simulink model "full_Model"  (R2023b)
settings: Solver=ode15s  StartTime=0.0  StopTime=200  RelTol=1e-3
InitFcn:
  | clear all
  | clc
  | 
  | load('EnvironmentData.mat')
  | load('userMap.mat')
  | 
  | starty = 1;
  | startx = 1;
  | endy = 20;
  | endx = 20;
  | objy = [];
  | objx = [];
  | bally = 11;
  | ballx = 11;
  | 
  | objPos=[objx,objy];
  | ballPos=[11,11,0.54];
  | boxPos=[];
  | 
  | ManipulatorSetup
  | init_quad_new_leg_raibert_strategy_v2
  | transitionMode = [-1];
values from neighbouring files (symbols this model uses):
  body = rigidBody('tool')    [InverseKinematicsV2.m]
  tar1Len = 9    [EnvironmentData.mat]
  target = [1 2.44274045536 4.0666557818 4.62742644863 6.44502800895 8.36141317519 9.41392894318 10.3865588461 10.4 10.4 11.7644392896 13.2870590067 ... (34 elements, 17x2)]    [EnvironmentData.mat]
  tarLen = 17    [EnvironmentData.mat]
undefined symbols (not defined in the file or in its folder): planner
libraries: sim3dlib x33, sharedtransform x2, visionsinks x1, visionanalysis x1, visiongeotforms x1, sim3dcameralib x1
(part 3 of 7)

== stateflow chart full_Model/Controller/High Level Mode Stateflow ==
  state ResetPos
    mode=0;
    ManipTask=1;
  state Stationary
    mode=0;
    ManipTask=0;
  state Turning_Right
    mode=2;
  state Walking
    mode=1;
  state Turning_Left
    mode=3;
  Turning_Right -> ResetPos [order 2] : [resetPos==1]{pos_index=pos_index+2}
  Stationary -> ResetPos [order 2] : [resetPos==1]{pos_index=pos_index+2}
  ResetPos -> Stationary : [manipState==5]
  Walking -> ResetPos [order 4] : [resetPos==1]{pos_index=pos_index+2}
  Turning_Left -> ResetPos [order 2] : [resetPos==1]{pos_index=pos_index+2}
  (default) -> Stationary : {pos_index =2 }
  Turning_Left -> Stationary [order 1] : [delta_theta < ang_threshold]
  Turning_Right -> Stationary [order 1] : [delta_theta > -ang_threshold]
  Stationary -> Walking [order 1] : [~target_reached]
  Walking -> Stationary [order 3] : [target_reached]
      | {pos_index = pos_index + 1}
  Walking -> Turning_Right [order 2] : [delta_theta < -ang_threshold]
  Walking -> Turning_Left [order 1] : [delta_theta > ang_threshold]
  data: pos_index output =0; mode output =0; target_reached input; delta_theta input; ang_threshold local =0.2; resetPos input; ManipTask output; manipState input

== stateflow chart full_Model/Controller/Chart ==
  state PathFollowing
    resetPos=0;
  state ManipulatorTask
    resetPos=1;
  (default) -> PathFollowing
  PathFollowing -> ManipulatorTask : [pos_index==tar1Len]
  ManipulatorTask -> PathFollowing : [manipState==5]
  data: pos_index input; tar1Len input; resetPos output; manipState input

== matlab function full_Model/TNR Annotation ==
  data: Area input; bboxes input size=[20 4]; scores input size=[20  1]; In input; In output
function In = TNRAnnotation(Area, bboxes, scores, In)

if ~isempty(bboxes)
    In = insertObjectAnnotation(In, 'rectangle',bboxes,scores);
    
end
In = insertObjectAnnotation(In, 'rectangle',Area,'.');
end

== matlab function full_Model/TNR Annotation1 ==
  data: bboxes input size=[20 4]; Output output; Area input
function Output = VisionOutput(bboxes, Area)
bbheight = height(bboxes);
xmin = Area(1);
xmax = Area(1) + Area(3);
ymin = Area(2);




%% first if statement decides whether we need to turn on not 
if bbheight == 1 
    if ((bboxes(1,1) + (bboxes(1,3)/2))  > xmin && (bboxes(1,1) + (bboxes(1,3)/2)) < xmax  && (bboxes(1,2) + bboxes(1,4)) > ymin)
        Turn = 1;
    else
        Turn = 0;
    end
elseif bbheight == 2
     if ((bboxes(1,1) + (bboxes(1,3)/2))  > xmin && (bboxes(1,1) + (bboxes(1,3)/2)) < xmax  && (bboxes(1,2) + bboxes(1,4)) > ymin ) || ...
        ((bboxes(2,1) + (bboxes(2,3)/2))  > xmin && (bboxes(2,1) + (bboxes(2,3)/2)) < xmax  && (bboxes(2,2) + bboxes(2,4)) > ymin )
        Turn = 1;
     else
        Turn = 0;
     end
elseif bbheight == 3
    if ((bboxes(1,1) + (bboxes(1,3)/2))  > xmin && (bboxes(1,1) + (bboxes(1,3)/2)) < xmax  && (bboxes(1,2) + bboxes(1,4)) > ymin ) || ...
       ((bboxes(2,1) + (bboxes(2,3)/2))  > xmin && (bboxes(2,1) + (bboxes(2,3)/2)) < xmax  && (bboxes(2,2) + bboxes(2,4)) > ymin ) || ...
       ((bboxes(3,1) + (bboxes(3,3)/2))  > xmin && (bboxes(3,1) + (bboxes(3,3)/2)) < xmax  && (bboxes(3,2) + bboxes(3,4)) > ymin )
        Turn = 1;
    else
        Turn = 0;
    end
elseif bbheight == 4
    if ((bboxes(1,1) + (bboxes(1,3)/2))  > xmin && (bboxes(1,1) + (bboxes(1,3)/2)) < xmax  && (bboxes(1,2) + bboxes(1,4)) > ymin ) || ...
       ((bboxes(2,1) + (bboxes(2,3)/2))  > xmin && (bboxes(2,1) + (bboxes(2,3)/2)) < xmax  && (bboxes(2,2) + bboxes(2,4)) > ymin ) || ...
       ((bboxes(3,1) + (bboxes(3,3)/2))  > xmin && (bboxes(3,1) + (bboxes(3,3)/2)) < xmax  && (bboxes(3,2) + bboxes(3,4)) > ymin ) || ...
       ((bboxes(4,1) + (bboxes(4,3)/2))  > xmin && (bboxes(4,1) + (bboxes(4,3)/2)) < xmax  && (bboxes(4,2) + bboxes(4,4)) > ymin )
        Turn = 1;
    else
        Turn = 0;
    end
elseif bbheight == 5    
    if ((bboxes(1,1) + (bboxes(1,3)/2))  > xmin && (bboxes(1,1) + (bboxes(1,3)/2)) < xmax  && (bboxes(1,2) + bboxes(1,4)) > ymin ) || ...
       ((bboxes(2,1) + (bboxes(2,3)/2))  > xmin && (bboxes(2,1) + (bboxes(2,3)/2)) < xmax  && (bboxes(2,2) + bboxes(2,4)) > ymin ) || ...
       ((bboxes(3,1) + (bboxes(3,3)/2))  > xmin && (bboxes(3,1) + (bboxes(3,3)/2)) < xmax  && (bboxes(3,2) + bboxes(3,4)) > ymin ) || ...
       ((bboxes(4,1) + (bboxes(4,3)/2))  > xmin && (bboxes(4,1) + (bboxes(4,3)/2)) < xmax  && (bboxes(4,2) + bboxes(4,4)) > ymin ) || ...
       ((bboxes(5,1) + (bboxes(5,3)/2))  > xmin && (bboxes(5,1) + (bboxes(5,3)/2)) < xmax  && (bboxes(5,2) + bboxes(5,4)) > ymin )
        Turn = 1 ;
    else
        Turn = 0 ;
    end
else
    Turn = 0;
end
%% next statement decideshow many objects are to the left and right of the viewpoint
left = 0;
right = 0;

if Turn == 0
    Output = 1;
elseif Turn == 1
    for i = 1:1:bbheight
        if (bboxes(i,1) + (bboxes(i,3)/2)) < 112
            left = left + 1;
        elseif (bboxes(i,1) + (bboxes(i,3)/2)) >= 112
            right = right + 1;
        else
            Output = 1;
        end

    end
else
    Output = 0;
end
%% final statemnet suggests which way to turn
if Turn == 1 && left >= right
    Output = 3;
elseif Turn == 1 && left < right
    Output = 2;
else
    Output = 1;
end

== matlab function full_Model/Balancing ==
  data: FLpos input; y output; FRpos input; RLpos input; RRpos input; FLang input; FRang input; RLang input; RRang input; linkLen input; linkWeight input; footStates input
function y = balancing(FLpos, FRpos, RLpos, RRpos, FLang, FRang, RLang, RRang, linkLen, linkWeight, footStates)

inputMatrix = [ % Input Parameters
    5, 3, 2, 78, 35, -4;   
    5, 9, 2, 85, 53, 1;   
    22, 3, 4, 78, 35, -4; 
    22, 9, 4, 85, 53, 1;  
    5, 5, 0, 0, 0, 4; ];

baseWeight = 10;
link_weight_per_length = 0.5;

combinedPositions = calculateAdjustedEndpoints(inputMatrix); % Calling Function
result = calculateMidpoints(combinedPositions, link_weight_per_length, baseWeight);
centerOfMass = calculateCenterOfMass(result);

intersect = checkPlaneIntersection(combinedPositions, inputMatrix, centerOfMass);
visualizePlaneAndLine(combinedPositions, inputMatrix, centerOfMass);

figure; hold on; colors = ['r', 'g', 'b', 'k'];


for i = 1:4 % Plotting individual positions
    positions = combinedPositions((i-1)*3+1:i*3, :);
    scatter3(positions(:, 1), positions(:, 2), positions(:, 3), 36, colors(i), 'filled');
    plot3(positions(:, 1), positions(:, 2), positions(:, 3), colors(i));
end

scatter3(centerOfMass(1),centerOfMass(2),centerOfMass(3));

% Plotting connecting lines using combinedPositions
plot3([combinedPositions(3, 1), combinedPositions(6, 1)], [combinedPositions(3, 2), combinedPositions(6, 2)], [combinedPositions(3, 3), combinedPositions(6, 3)], 'm--', 'LineWidth', 2);
plot3([combinedPositions(3, 1), combinedPositions(9, 1)], [combinedPositions(3, 2), combinedPositions(9, 2)], [combinedPositions(3, 3), combinedPositions(9, 3)], 'm--', 'LineWidth', 2);
plot3([combinedPositions(12, 1), combinedPositions(6, 1)], [combinedPositions(12, 2), combinedPositions(6, 2)], [combinedPositions(12, 3), combinedPositions(6, 3)], 'c--', 'LineWidth', 2);
plot3([combinedPositions(12, 1), combinedPositions(9, 1)], [combinedPositions(12, 2), combinedPositions(9, 2)], [combinedPositions(12, 3), combinedPositions(9, 3)], 'c--', 'LineWidth', 2);

xlabel('X'); ylabel('Y'); zlabel('Z'); 
title('3D Plot of Combined Positions'); 
axis equal; grid on; view(3); hold off;

end


%% Functions

function combinedPositions = calculateAdjustedEndpoints(inputMatrix)
    combinedPositions = zeros(12, 3); % Initialize the output matrix
    for i = 1:4
        % Extract input parameters
        Foot = inputMatrix(i, 1:3);
        Ankle_Angle = inputMatrix(i, 4);
        Knee_Angle = inputMatrix(i, 5);
        Shoulder_angle = inputMatrix(i, 6);
        Link1_Length = inputMatrix(5, 1);
        Link2_Length = inputMatrix(5, 2);
        % Calculate the endpoints
        Link1_endpoint = zeros(1, 3);
        Link2_endpoint = zeros(1, 3);
        Link1_endpoint(1) = Foot(1) + Link1_Length * cos(deg2rad(Ankle_Angle));
        Link1_endpoint(2) = Foot(2);
        Link1_endpoint(3) = Foot(3) + Link1_Length * sin(deg2rad(Ankle_Angle));
        Link2_endpoint(1) = Link1_endpoint(1) + Link2_Length * cos(deg2rad(Knee_Angle));
        Link2_endpoint(2) = Link1_endpoint(2);
        Link2_endpoint(3) = Link1_endpoint(3) + Link2_Length * sin(deg2rad(Knee_Angle));
        % Adjust the endpoints based on the shoulder angle
        theta = deg2rad(Shoulder_angle);
        R = [1 0 0; 0 cos(theta) -sin(theta); 0 sin(theta) cos(theta)];
        Link1_endpoint_adjusted = R * (Link1_endpoint - Foot).' + Foot.';
        Link2_endpoint_adjusted = R * (Link2_endpoint - Foot).' + Foot.';
        % Assign the calculated positions to the output matrix
        startPos = (i-1)*3 + 1;
        combinedPositions(startPos:startPos+2, :) = [Foot; Link1_endpoint_adjusted.'; Link2_endpoint_adjusted.'];
    end
end

function outputMatrix = calculateMidpoints(inputMatrix, link_weight_per_length, baseWeight)
    outputMatrix = zeros(9, 4);     % Initialize the output matrix
    pointPairs = [1, 2; 2, 3; 4, 5; 5, 6; 7, 8; 8, 9; 10, 11; 11, 12]; % Define the pair
    for i = 1:size(pointPairs, 1)   % Calculate midpoint pos and link weight for each pair
        point1 = inputMatrix(pointPairs(i, 1), :);
        point2 = inputMatrix(pointPairs(i, 2), :);
        midpoint = (point1 + point2) / 2;
        distance = sqrt(sum((point1 - point2) .^ 2));
        weight = distance * link_weight_per_length;
        outputMatrix(i, 1:3) = midpoint;
        outputMatrix(i, 4) = weight;
    end
    centerPoints = mean(inputMatrix([3, 6, 9, 12], :), 1);  % Calculate base center
    outputMatrix(9, :) = [centerPoints, baseWeight];        % Add the baseWeight as its mass
end

function centerOfMass = calculateCenterOfMass(inputMatrix)
    % Initialize the variables for the sum of weighted coordinates and total mass
    weightedSum = [0, 0, 0];
    totalMass = 0;
    % Loop through each point
    for i = 1:size(inputMatrix, 1)
        % Extract the current point's coordinates and mass
        x = inputMatrix(i, 1);
        y = inputMatrix(i, 2);
        z = inputMatrix(i, 3);
        mass = inputMatrix(i, 4);
        % Update the weighted sum and total mass
        weightedSum = weightedSum + [x, y, z] * mass;
        totalMass = totalMass + mass;
    end
    % Calculate the center of mass coordinates
    centerOfMassCoordinates = weightedSum / totalMass;
    % Combine the center of mass coordinates with the total mass
    centerOfMass = [centerOfMassCoordinates, totalMass];
end

function intersect = checkPlaneIntersection(combinedPositions, inputMatrix, centerOfMass)
    % Determine which points to use from the combinedPositions matrix
    switch inputMatrix(5,6)
        case 1
            points = combinedPositions([6, 9, 12], :);
        case 2
            points = combinedPositions([3, 9, 12], :);
        case 3
            points = combinedPositions([3, 6, 12], :);
        case 4
            points = combinedPositions([3, 6, 9], :);
        otherwise
            error('Invalid input in inputMatrix(5,6)');
    end

    % Calculate the plane equation coefficients
    p1 = points(1, :);
    p2 = points(2, :);
    p3 = points(3, :);
    normal = cross(p2 - p1, p3 - p1);
    A = normal(1);
    B = normal(2);
    C = normal(3);
    D = -dot(normal, p1);

    % Check if the line from centerOfMass intersects the plane
    x0 = centerOfMass(1);
    y0 = centerOfMass(2);

    % If C is zero, the plane is parallel to the z-axis and can't intersect
    if C == 0
        intersect = 'NO';
        return;
    end

    % Find intersection point on the plane
    t = -(A * x0 + B * y0 + D) / C;
    intersectionPoint = [x0, y0, t];

    % Check if the intersection point is inside the triangle
    if isPointInTriangle(intersectionPoint, p1, p2, p3)
        intersect = 'YES';
    else
        intersect = 'NO';
    end
end

function inside = isPointInTriangle(pt, v1, v2, v3)
    % Barycentric coordinate system
    dX = pt(1) - v3(1);
    dY = pt(2) - v3(2);
    dX21 = v2(1) - v1(1);
    dY12 = v1(2) - v2(2);
    D = dY12 * (v3(1) - v1(1)) + dX21 * (v3(2) - v1(2));
    s = dY12 * dX + dX21 * dY;
    t = (v3(2) - v1(2)) * dX + (v1(1) - v3(1)) * dY;
    
    if D < 0
        inside = s <= 0 && t <= 0 && s + t >= D;
    else
        inside = s >= 0 && t >= 0 && s + t <= D;
    end
end


function visualizePlaneAndLine(combinedPositions, inputMatrix, centerOfMass)
    % Select points based on inputMatrix value
    switch inputMatrix(5,6)
        case 1
            points = combinedPositions([6, 9, 12], :);
        case 2
            points = combinedPositions([3, 9, 12], :);
        case 3
            points = combinedPositions([3, 6, 12], :);
        case 4
            points = combinedPositions([3, 6, 9], :);
        otherwise
            error('Invalid input in inputMatrix(5,6)');
    end

    % Plane calculation
    normal = cross(points(2,:) - points(1,:), points(3,:) - points(1,:));
    point = points(1,:);
    [xGrid, yGrid] = meshgrid(linspace(min(combinedPositions(:,1)), max(combinedPositions(:,1)), 10), ...
                             linspace(min(combinedPositions(:,2)), max(combinedPositions(:,2)), 10));
    zGrid = (-normal(1) * (xGrid - point(1)) - normal(2) * (yGrid - point(2)))/normal(3) + point(3);

    % Line calculation
    lineZ = linspace(min(zGrid(:)), max(zGrid(:)), 100);
    lineX = centerOfMass(1) * ones(size(lineZ));
    lineY = centerOfMass(2) * ones(size(lineZ));

    % Plotting
    figure;
    hold on;
    surf(xGrid, yGrid, zGrid, 'FaceAlpha', 0.5); % Draw plane
    plot3(lineX, lineY, lineZ, 'r', 'LineWidth', 2); % Draw line
    plot3(points(:,1), points(:,2), points(:,3), 'ko', 'MarkerSize', 10, 'MarkerFaceColor', 'k'); % Draw points
    xlabel('X');
    ylabel('Y');
    zlabel('Z');
    title('Visualization of Plane and Line');
    grid on;
    view(3);

    y = 0;
end

== matlab function full_Model/Controller/MATLAB Function1 ==
  settings: updateMethod=DISCRETE
  data: go input; mode output; targets input; tar1Len input; tarLen input; x input; y input; angle input; done output
function [mode,done] = broadside(go,targets,tar1Len,tarLen,x,y,angle)

persistent targetAssigned
if isempty(targetAssigned)
    targetAssigned=0;
end

persistent broadTarget
if isempty(broadTarget)
    broadTarget=[0,0];
end

persistent points
if isempty(points)
    points=0;
end

persistent point1
if isempty(point1)
    point1=[0,0];
end

persistent point2
if isempty(point2)
    point2=[0,0];
end

persistent currentTarget
if isempty(currentTarget)
    currentTarget=[0,0];
end


if go==1||go==2
    if targetAssigned==0
        if go==1
            broadTarget=targets(tar1Len,:);
        elseif go==2
            broadTarget=targets(tarLen,:);
        end
        if y>broadTarget(2)
            spacing=1;
        else
            spacing=-1;
        end
        if x>broadTarget(1)
            points=2;
            point1=[x,broadTarget(2)+spacing];
            point2=[broadTarget(1),broadTarget(2)+spacing];
        else
            points=1;
            point1=[broadTarget(1),broadTarget(2)+spacing];
        end
        currentTarget=point1;
        targetAssigned=1;
    end
    delta=currentTarget-[x,y];
    deltaDist=sqrt(delta(1).^2+delta(2).^2);
    targetAngle=atan2(delta(2),delta(1));
    deltaAngle=targetAngle-angle;
    if abs(deltaDist)>=0.2
        if deltaAngle<-0.1
            %disp('im left')
            %turn right
            mode=2;

        elseif deltaAngle>0.1
            %disp('im right')
            %turn left
            mode=3;
        else
            %disp('im forward')
            mode=1;
        end
        done=0;
    else
        if (currentTarget-point1)*[1;1]==0&&points==1
            currentTarget=[broadTarget(1),broadTarget(2)];
            done=0;
        elseif (currentTarget-point1)*[1;1]==0&&points==2
            currentTarget=point2;
            done=0;
        elseif (currentTarget-point2)*[1;1]==0
            currentTarget=[broadTarget(1),broadTarget(2)];
            done=0;
        else
            done=1;
        end
        mode=0;
    end
else
    targetAssigned=0;
    done=0;
    mode=0;
end

== stateflow chart full_Model/Controller/Task Controller/Task Controller Stateflow ==
  state PathFollowing
    endSim=false;
    resetPos=0;
    sqrt((target(tar1Len,1)-x).^2+ (target(tar1Len,2)-y).^2);
  state ManipulatorTask1
    resetPos=1;
  state PathFollowing2
    resetPos=0;
    sqrt((target(tar1Len,1)-x).^2+ (target(tar1Len,2)-y).^2);
  state ManipulatorTask2
    resetPos=2;
  state EndSim
    resetPos=0;
    endSim=true;
  PathFollowing -> ManipulatorTask1 : [sqrt((target(tar1Len,1)-x).^2+(target(tar1Len,2)-y).^2)<=1.5]{posToSkip=tar1Len-pos_index}
  (default) -> PathFollowing
  ManipulatorTask1 -> PathFollowing2 : [manipState>=5]
  PathFollowing2 -> ManipulatorTask2 : [sqrt((target(tarLen,1)-x).^2+ (target(tarLen,2)-y).^2)<=1.5]
  ManipulatorTask2 -> EndSim : [manipState>=11]
  data: tar1Len input; resetPos output; manipState input; tarLen input; endSim output; target input; y input; posToSkip output; x input; pos_index input

== stateflow chart full_Model/Controller/Path follower stateflow ==
  state Stationary1
    mode=0;
  state Walking1
    mode=1;
  state Turning_Left1
    mode=1;
  note: 0.35
  note: 1
  state ManipTask1
    ManipTask=1;
  state Broadside
    broadside=1;
  state Stationary
    mode=0;
  state ResetPos1
    mode=0;
  state Turning_Right
    mode=2;
  state Turning_Left
    mode=3;
  state Walking
    mode=1;
  state ManipTask2
    ManipTask=2;
  state ResetPos2
    mode=0;
  state Broadside1
    broadside=2;
  Walking1 -> Turning_Left1 : [delta_theta < ang_threshold]
  Stationary1 -> Walking1 : [~target_reached]
  (default) -> Stationary1 : {pos_index =2;bodyMode=0}
  Broadside -> ManipTask1 : [broadFinished==1&&stopped]{broadside=0}
  Stationary -> Stationary [order 3] : [target_reached&&pos_index~=tarLen]
      | {pos_index = pos_index + 1}
  ManipTask1 -> Stationary : [resetPos==0]
  Stationary -> ResetPos1 [order 1] : [resetPos==1]
  Stationary -> ResetPos2 [order 4] : [resetPos==2]
  Turning_Left -> Stationary [order 1] : [delta_theta < ang_threshold]
  Turning_Right -> Stationary [order 1] : [delta_theta > -ang_threshold]
  Walking -> Stationary [order 1] : [target_reached&&pos_index~=tarLen]
      | {pos_index = pos_index + 1}
  Stationary -> Walking [order 2] : [~target_reached]
  Turning_Right -> ResetPos1 [order 2] : [resetPos==1]
  Walking -> Turning_Left [order 2] : [delta_theta > ang_threshold]
  Turning_Left -> ResetPos1 [order 3] : [resetPos==1]
  Walking -> ResetPos1 [order 5] : [resetPos==1]
  Turning_Left -> ResetPos2 [order 2] : [resetPos==2]
  Turning_Right -> ResetPos2 [order 3] : [resetPos==2]
  Walking -> Turning_Right [order 4] : [delta_theta < -ang_threshold]
  Broadside1 -> ManipTask2 : [broadFinished==1&&stopped]{broadside=0}
  Walking -> ResetPos2 [order 3] : [resetPos==2]
  ResetPos2 -> Broadside1 : [stopped]
  data: pos_index output =0; mode output =0; target_reached input; delta_theta input; ang_threshold local =0.2; resetPos input; ManipTask output; stopped input; bodyMode output; tarLen input; broadside output; broadFinished input; posToSkip input

== matlab function full_Model/UE INPUT /Euler to Matrix ==
  data: EulAngles input; Matrix output
function Matrix = fcn(EulAngles)

Matrix = eul2rotm(EulAngles);

== matlab function full_Model/UE INPUT /Matrix to AxisAngle ==
  data: Matrix input; AxisAngle output
function AxisAngle = fcn(Matrix)

AxisAngle = rotm2axang(Matrix);
